simulink library "csg"  (Simulink 8.1)
settings: Solver=ode1  StartTime=0.0  StopTime=Inf  FixedStep=0.001  RelTol=1e-3
PostLoadFcn:
  | , if any(exist('dsrtsu_mdlpostloadfcn', 'file') == [2, 3, 6]), try dsrtsu_mdlpostloadfcn('Execute', bdroot); catch fprintf('Error in PostLoadFcn (dsrtsu_mdlpostloadfcn) for model "%s":\n %s\n', bdroot, lasterr); end, end,
undefined symbols (not defined in the file or in its folder): KACC_SteadyTGapPTCMargin_m
settings Model: DSRTSU_INTERNAL_RTI_VER=450  DSRTSU_INTERNAL_RTI_TYPE=rti1401  Creator=idiada  LastModifiedBy=idiada

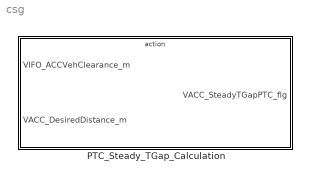
== system csg ==
  PTC_Steady_TGap_Calculation : Subsystem  TreatAsAtomicUnit=on

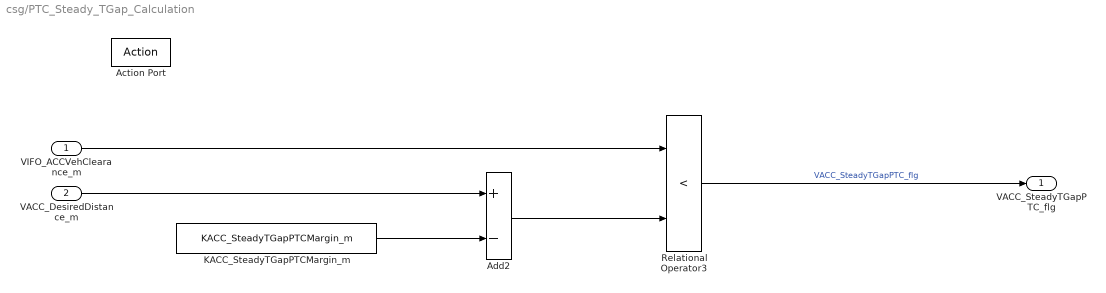
== system csg/PTC_Steady_TGap_Calculation ==
  VIFO_ACCVehClearance_m : Inport
  VACC_DesiredDistance_m : Inport  Port=2
  Action Port : ActionPort
  Add2 : Sum  Inputs=+-
  KACC_SteadyTGapPTCMargin_m : Constant  Value=KACC_SteadyTGapPTCMargin_m
  Relational Operator3 : RelationalOperator  Operator=<  OutDataTypeStr=boolean
  VACC_SteadyTGapPTC_flg : Outport
  wires:
  VACC_DesiredDistance_m/1 -> Add2/1
  VIFO_ACCVehClearance_m/1 -> Relational Operator3/1
  Add2/1 -> Relational Operator3/2
  KACC_SteadyTGapPTCMargin_m/1 -> Add2/2
  Relational Operator3/1 -> VACC_SteadyTGapPTC_flg/1  "VACC_SteadyTGapPTC_flg"
